simulink model "windmi_8"  (Simulink 7.7)
settings: Solver=ode15s  StartTime=0.0  StopTime=86400*3  RelTol=1e-4
values from neighbouring files (symbols this model uses):
  A = (L1*L-M^2)^(-1)    (= 0.000277778549385)    [windmi.m]
  A_eff = 2*(R_Earth^2)    (= 81408800000000)    [windmi.m]
  alpha = 7.550246e+11    (= 755024600000)    [windmi.m]
  B_tr = 5e-9    (= 5e-09)    [windmi.m]
  beta = 1.1    [windmi.m]
  C = 8000    [windmi.m]
  C1 = 500    [windmi.m]
  Ic = 2e7    (= 20000000)    [windmi.m]
  inv_dI = (del_I)^(-1)    (= 8e-06)    [windmi.m]
  L = 90    [windmi.m]
  L1 = 40    [windmi.m]
  L2 = 8    [windmi.m]
  L_y = 5*R_Earth    (= 31900000)    [windmi.m]
  M = 0.1    [windmi.m]
  mu0 = 4.2e-9    (= 4.2e-09)    [windmi.m]
  Omega = 10000*R_Earth^3    (= 2.59694072e+24)    [windmi.m]
  R_A2 = 0.3    [windmi.m]
  R_prc = 0.1    [windmi.m]
  Sigma = 5    [windmi.m]
  SigmaI = 3    [windmi.m]
  t_delay = 35    [Electron_Energization_Index_v3_0_parameters.m]    (also in windmi.m = -(250*6380)/mean(1.0*Vx))
  tau_rc = 12*3600    (= 43200)    [windmi.m]
  tauE = 1*3600    (= 3600)    [windmi.m]
  taup = 0.01*600    (= 6)    [windmi.m]
settings Model: Creator=espencer  LastModifiedBy=edmund  ExtModeAutoUpdateStatusClock=off  TunableVars=A,A_eff,B_tr,C,C1,Ic,L,L1,L2,L_y,M,Omega,R_A2,R_prc,Sigma,SigmaI,alpha,alpha_F,beta,inv_dI,mu0,tauE,tau_rc,taup  TunableVarsStorageClass=Auto,Auto,Auto,Auto,Auto,Auto,Auto,Auto,Auto,Auto,Auto,Auto,Auto,Auto,Auto,Auto,Auto,Auto,Auto,Auto,Auto,Auto,Auto,Auto  TunableVarsTypeQualifier=,,,,,,,,,,,,,,,,,,,,,,,  BufferReuse=off
settings SolverCC: MaxConsecutiveZCs=10e6
settings DataIOCC: LimitDataPoints=off
settings OptimizationCC: BlockReduction=off  BooleanDataType=off  InlineParams=on  OptimizeBlockIOStorage=off  BufferReuse=off  ExpressionFolding=off  LocalBlockOutputs=off  InitFltsAndDblsToZero=on
settings DebuggingCC: SaveWithParameterizedLinksMsg=none  SignalResolutionControl=TryResolveAllWithWarning  SolverPrmCheckMsg=none  MultiTaskDSMMsg=warning  MultiTaskCondExecSysMsg=none  StrictBusMsg=None
settings HardwareCC: TargetUnknown=on
settings RTWCC: IncludeERTFirstTime=on
settings GRTTargetCC: TargetFcnLib=ansi_tfl_tmw.mat

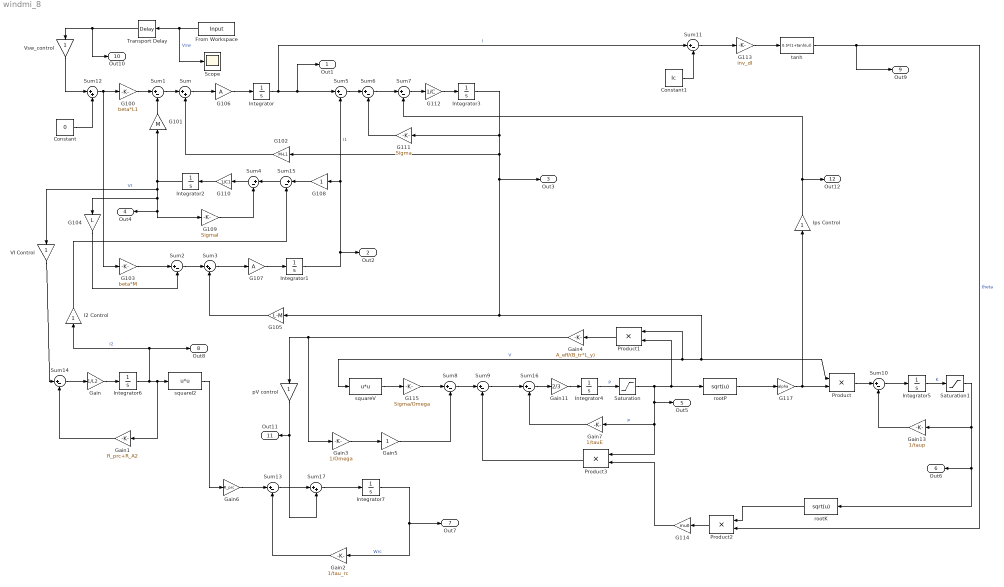
== system windmi_8 ==
  Constant : Constant  Value=0
  Constant1 : Constant  Value=Ic
  From Workspace : FromWorkspace  VariableName=Input  SampleTime=0
  G100 : Gain  Gain=beta*L1  SaturateOnIntegerOverflow=on  OutDataTypeStr=Inherit: Same as input  ParamDataTypeStr=Inherit: Same as input
  G101 : Gain  Gain=M  SaturateOnIntegerOverflow=on  OutDataTypeStr=Inherit: Same as input  ParamDataTypeStr=Inherit: Same as input
  G102 : Gain  Gain=M-L1  SaturateOnIntegerOverflow=on  OutDataTypeStr=Inherit: Same as input  ParamDataTypeStr=Inherit: Same as input
  G103 : Gain  Gain=beta*M  SaturateOnIntegerOverflow=on  OutDataTypeStr=Inherit: Same as input  ParamDataTypeStr=Inherit: Same as input
  G104 : Gain  Gain=L  SaturateOnIntegerOverflow=on  OutDataTypeStr=Inherit: Same as input  ParamDataTypeStr=Inherit: Same as input
  G105 : Gain  Gain=L-M  SaturateOnIntegerOverflow=on  OutDataTypeStr=Inherit: Same as input  ParamDataTypeStr=Inherit: Same as input
  G106 : Gain  Gain=A  SaturateOnIntegerOverflow=on  OutDataTypeStr=Inherit: Same as input  ParamDataTypeStr=Inherit: Same as input
  G107 : Gain  Gain=A  SaturateOnIntegerOverflow=on  OutDataTypeStr=Inherit: Same as input  ParamDataTypeStr=Inherit: Same as input
  G108 : Gain  SaturateOnIntegerOverflow=on  OutDataTypeStr=Inherit: Same as input  ParamDataTypeStr=Inherit: Same as input
  G109 : Gain  Gain=SigmaI  SaturateOnIntegerOverflow=on  OutDataTypeStr=Inherit: Same as input  ParamDataTypeStr=Inherit: Same as input
  G110 : Gain  Gain=1/C1  SaturateOnIntegerOverflow=on  OutDataTypeStr=Inherit: Same as input  ParamDataTypeStr=Inherit: Same as input
  G111 : Gain  Gain=Sigma  SaturateOnIntegerOverflow=on  OutDataTypeStr=Inherit: Same as input  ParamDataTypeStr=Inherit: Same as input
  G112 : Gain  Gain=1/C  SaturateOnIntegerOverflow=on  OutDataTypeStr=Inherit: Same as input  ParamDataTypeStr=Inherit: Same as input
  G113 : Gain  Gain=inv_dI  SaturateOnIntegerOverflow=on  OutDataTypeStr=Inherit: Same as input  ParamDataTypeStr=Inherit: Same as input
  G114 : Gain  Gain=mu0  SaturateOnIntegerOverflow=on  OutDataTypeStr=Inherit: Same as input  ParamDataTypeStr=Inherit: Same as input
  G115 : Gain  Gain=Sigma/Omega  SaturateOnIntegerOverflow=on  OutDataTypeStr=Inherit: Same as input  ParamDataTypeStr=Inherit: Same as input
  G117 : Gain  Gain=alpha  SaturateOnIntegerOverflow=on  OutDataTypeStr=Inherit: Same as input  ParamDataTypeStr=Inherit: Same as input
  Gain : Gain  Gain=1/L2  SaturateOnIntegerOverflow=on  OutDataTypeStr=Inherit: Same as input  ParamDataTypeStr=Inherit: Same as input
  Gain1 : Gain  Gain=R_prc+R_A2  SaturateOnIntegerOverflow=on  OutDataTypeStr=Inherit: Same as input  ParamDataTypeStr=Inherit: Same as input
  Gain11 : Gain  Gain=2/3  SaturateOnIntegerOverflow=on  OutDataTypeStr=Inherit: Same as input  ParamDataTypeStr=Inherit: Same as input
  Gain13 : Gain  Gain=1/taup  SaturateOnIntegerOverflow=on  OutDataTypeStr=Inherit: Same as input  ParamDataTypeStr=Inherit: Same as input
  Gain2 : Gain  Gain=1/tau_rc  SaturateOnIntegerOverflow=on  OutDataTypeStr=Inherit: Same as input  ParamDataTypeStr=Inherit: Same as input
  Gain3 : Gain  Gain=1/Omega  SaturateOnIntegerOverflow=on  OutDataTypeStr=Inherit: Same as input  ParamDataTypeStr=Inherit: Same as input
  Gain4 : Gain  Gain=A_eff/(B_tr*L_y)  SaturateOnIntegerOverflow=on  OutDataTypeStr=Inherit: Same as input  ParamDataTypeStr=Inherit: Same as input
  Gain5 : Gain  SaturateOnIntegerOverflow=on  OutDataTypeStr=Inherit: Same as input  ParamDataTypeStr=Inherit: Same as input
  Gain6 : Gain  Gain=R_prc  SaturateOnIntegerOverflow=on  OutDataTypeStr=Inherit: Same as input  ParamDataTypeStr=Inherit: Same as input
  Gain7 : Gain  Gain=1/tauE  SaturateOnIntegerOverflow=on  OutDataTypeStr=Inherit: Same as input  ParamDataTypeStr=Inherit: Same as input
  I2 Control : Gain  SaturateOnIntegerOverflow=on  OutDataTypeStr=Inherit: Same as input  ParamDataTypeStr=Inherit: Same as input
  Integrator{,1..7} (8 alike) : Integrator
  Ips Control : Gain  SaturateOnIntegerOverflow=on  OutDataTypeStr=Inherit: Same as input  ParamDataTypeStr=Inherit: Same as input
  Product{,1..3} (4 alike) : Product  SaturateOnIntegerOverflow=on  RndMeth=Zero  InputSameDT=on  OutDataTypeStr=Inherit: Same as first input
  Saturation : Saturate  UpperLimit=1  LowerLimit=1e-24
  Saturation1 : Saturate  UpperLimit=1e32  LowerLimit=1e-15
  Scope : Scope
  Sum{,3,12,17} (4 alike) : Sum  Inputs=|++  SaturateOnIntegerOverflow=on  InputSameDT=on  OutDataTypeStr=Inherit: Same as first input
  Sum{1..2,4..11,13..16} (14 alike) : Sum  Inputs=|+-  SaturateOnIntegerOverflow=on  InputSameDT=on  OutDataTypeStr=Inherit: Same as first input
  Transport Delay : TransportDelay  DelayTime=t_delay  BufferSize=4096
  VI Control : Gain  SaturateOnIntegerOverflow=on  OutDataTypeStr=Inherit: Same as input  ParamDataTypeStr=Inherit: Same as input
  Vsw_control : Gain  SaturateOnIntegerOverflow=on  OutDataTypeStr=Inherit: Same as input  ParamDataTypeStr=Inherit: Same as input
  pV control : Gain  SaturateOnIntegerOverflow=on  OutDataTypeStr=Inherit: Same as input  ParamDataTypeStr=Inherit: Same as input
  rootK : Fcn  Expr=sqrt(u)
  rootP : Fcn  Expr=sqrt(u)
  squareI2 : Fcn  Expr=u*u
  squareV : Fcn  Expr=u*u
  tanh : Fcn  Expr=0.5*(1+tanh(u))
  Out1 : Outport
  Out2 : Outport  Port=2
  Out3 : Outport  Port=3
  Out4 : Outport  Port=4
  Out5 : Outport  Port=5
  Out6 : Outport  Port=6
  Out7 : Outport  Port=7
  Out8 : Outport  Port=8
  Out9 : Outport  Port=9
  Out10 : Outport  Port=10
  Out11 : Outport  Port=11
  Out12 : Outport  Port=12
  wires:
  Sum1/1 -> Sum/1
  G103/1 -> Sum2/1
  Sum2/1 -> Sum3/1
  Integrator2/1 -> G104/1, G109/1, Out4/1, VI Control/1, G101/1  "VI"
  G109/1 -> Sum4/2
  Integrator1/1 -> Out2/1, G108/1, Sum5/2  "I1"
  G101/1 -> Sum1/2
  G104/1 -> Sum2/2
  Integrator/1 -> Sum11/1, Sum5/1, Out1/1  "I"
  Sum5/1 -> Sum6/1
  Sum6/1 -> Sum7/1
  Sum7/1 -> G112/1
  G112/1 -> Integrator3/1
  Integrator3/1 -> G111/1, G102/1, Product/1, squareV/1, Product1/1, G105/1, Out3/1  "V"
  G111/1 -> Sum6/2
  G102/1 -> Sum/2
  G105/1 -> Sum3/2
  squareV/1 -> G115/1
  G115/1 -> Sum8/1
  Sum8/1 -> Sum9/1
  Gain11/1 -> Integrator4/1
  Integrator4/1 -> Saturation/1  "P"
  rootP/1 -> G117/1
  Sum10/1 -> Integrator5/1
  Gain13/1 -> Sum10/2
  Product/1 -> Sum10/1
  Constant1/1 -> Sum11/2
  Sum11/1 -> G113/1
  G113/1 -> tanh/1
  G106/1 -> Integrator/1
  Sum/1 -> G106/1
  G100/1 -> Sum1/1
  Sum3/1 -> G107/1
  G107/1 -> Integrator1/1
  Sum4/1 -> G110/1
  G110/1 -> Integrator2/1
  Ips Control/1 -> Sum7/2, Out12/1
  Sum12/1 -> G100/1, G103/1
  Product1/1 -> Gain4/1
  Sum14/1 -> Gain/1
  Gain/1 -> Integrator6/1
  Integrator6/1 -> Gain1/1, squareI2/1, I2 Control/1, Out8/1  "I2"
  Gain1/1 -> Sum14/2
  Sum15/1 -> Sum4/1
  G108/1 -> Sum15/1
  squareI2/1 -> Gain6/1
  Gain6/1 -> Sum13/1
  Sum13/1 -> Sum17/1
  Sum17/1 -> Integrator7/1
  Integrator7/1 -> Gain2/1, Out7/1  "Wrc"
  Gain2/1 -> Sum13/2
  Product3/1 -> Sum9/2
  tanh/1 -> Product2/2, Out9/1  "theta"
  G114/1 -> Product3/2
  Gain3/1 -> Gain5/1
  Gain5/1 -> Sum8/2
  Gain7/1 -> Sum16/2
  Sum9/1 -> Sum16/1
  Sum16/1 -> Gain11/1
  Gain4/1 -> Gain3/1, pV control/1
  I2 Control/1 -> Sum15/2
  VI Control/1 -> Sum14/1
  pV control/1 -> Sum17/2, Out11/1
  Product2/1 -> G114/1
  Constant/1 -> Sum12/2
  G117/1 -> Product/2, Ips Control/1
  rootK/1 -> Product2/1
  From Workspace/1 -> Transport Delay/1, Scope/1  "Vsw"
  Saturation/1 -> Product1/2, rootP/1, Product3/1, Gain7/1, Out5/1  "P"
  Integrator5/1 -> Saturation1/1  "K"
  Saturation1/1 -> Gain13/1, rootK/1, Out6/1
  Transport Delay/1 -> Vsw_control/1, Out10/1
  Vsw_control/1 -> Sum12/1
